simulink model "DcMotorLeadController"  (R2017a)
settings: Solver=ode45  StartTime=0.0  StopTime=3  MaxStep=0.001  RelTol=1e-3
values from neighbouring files (symbols this model uses):
  Ka = Kc*tz/tp    (= 18.4615384615)    [lab6Scrypt.m]
  Kmot = Kamp*Kpot*K    (= 71.6197243914)    [lab6Scrypt.m]
  P = 1/tp    (= 120)    [lab6Scrypt.m]
  tau = 0.2    [lab6Scrypt.m]
  Z = 1/tz    (= 13)    [lab6Scrypt.m]
settings Model: Creator=hernandezmarvinalexander  LastModifiedBy=maherna4

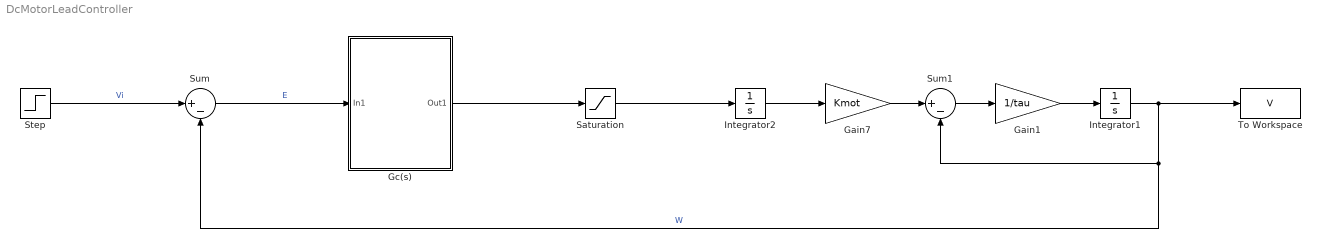
== system DcMotorLeadController ==
  Gain1 : Gain  Gain=1/tau
  Gain7 : Gain  Gain=Kmot
  Gc(s) : Subsystem
  Integrator1 : Integrator
  Integrator2 : Integrator
  Saturation : Saturate  UpperLimit=10  LowerLimit=-10
  Step : Step  Time=0  After=50  SampleTime=0
  Sum : Sum  Inputs=|+-
  Sum1 : Sum  Inputs=|+-
  To Workspace : ToWorkspace  VariableName=V  SampleTime=-1
  wires:
  Sum/1 -> Gc(s)/1(In1)  "E"
  Step/1 -> Sum/1  "Vi"
  Integrator2/1 -> Gain7/1
  Integrator1/1 -> Sum/2, Sum1/2, To Workspace/1  "W"
  Gain1/1 -> Integrator1/1
  Gain7/1 -> Sum1/1
  Sum1/1 -> Gain1/1
  Saturation/1 -> Integrator2/1
  Gc(s)/1(Out1) -> Saturation/1

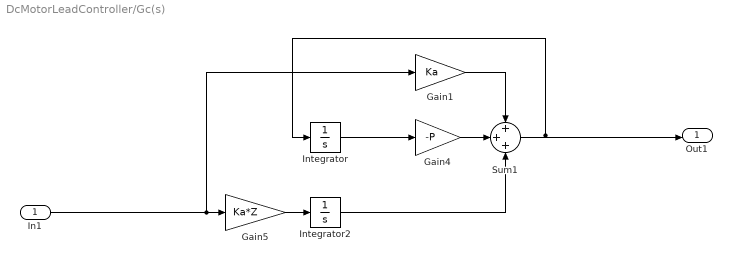
== system DcMotorLeadController/Gc(s) ==
  In1 : Inport
  Gain1 : Gain  Gain=Ka
  Gain4 : Gain  Gain=-P
  Gain5 : Gain  Gain=Ka*Z
  Integrator : Integrator
  Integrator2 : Integrator
  Sum1 : Sum  Inputs=+++
  Out1 : Outport
  wires:
  Gain4/1 -> Sum1/2
  Gain1/1 -> Sum1/1
  Sum1/1 -> Out1/1, Integrator/1
  Integrator2/1 -> Sum1/3
  Gain5/1 -> Integrator2/1
  In1/1 -> Gain1/1, Gain5/1
  Integrator/1 -> Gain4/1
